simulink library "nodeNetBuoyForce_ul"  (R2020a)
settings: Solver=VariableStepAuto  StartTime=0.0  StopTime=10.0  RelTol=1e-3
settings Model: Creator=mcobb  LastModifiedBy=andre
settings DataIOCC: ReturnWorkspaceOutputs=off
settings DebuggingCC: ArithmeticOperatorsInVariantConditions=warning
settings SFSimCC: CustomCodeUndefinedFunction=UseInterfaceOnly

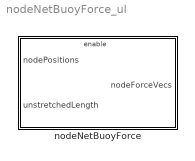
== system nodeNetBuoyForce_ul ==
  nodeNetBuoyForce : Subsystem  mask{fluidDensity=0, tetherDensity=0, diameter=0, gravity=0}
      mask prompts: fluidDensity "Fluid density"; tetherDensity "Tether density"; diameter "Tether diameter"; gravity "Gravitational acceleration"
      settings: MinAlgLoopOccurrences=on

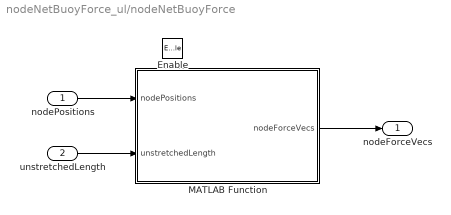
== system nodeNetBuoyForce_ul/nodeNetBuoyForce ==
  nodePositions : Inport
  unstretchedLength : Inport  Port=2
  Enable : EnablePort
  MATLAB Function : MATLAB Function  TreatAsAtomicUnit=on
  nodeForceVecs : Outport  VectorParamsAs1DForOutWhenUnconnected=off
  wires:
  MATLAB Function/1(nodeForceVecs) -> nodeForceVecs/1
  nodePositions/1 -> MATLAB Function/1(nodePositions)
  unstretchedLength/1 -> MATLAB Function/2(unstretchedLength)

== matlab function nodeNetBuoyForce_ul/nodeNetBuoyForce/MATLAB Function ==
  data: nodePositions input; unstretchedLength input; nodeForceVecs output; tetherDensity parameter; fluidDensity parameter; diameter parameter; gravity parameter
function nodeForceVecs  = fcn(...
    nodePositions,unstretchedLength,...
    tetherDensity, fluidDensity, diameter, gravity)

% In this notation, N is the number of nodes

% Length of each link 1xN-1
linkLengths = sqrt(sum(diff(nodePositions,1,2).^2));

% Total length of all links, assuming they're straight lines, scalar
numericalTotalLength = sum(linkLengths);

% Number of links, scalar
numLinks = size(linkLengths,2);

% Total volume based on unspooled length, scalar
analyticalTotalVol  = sum(unstretchedLength)*(pi/4)*diameter^2;

% Total mass, based on unspooled length, scalar
analyticalTotalMass = tetherDensity*analyticalTotalVol;

% Mass of each link, 1xN-1
linkMasses  = analyticalTotalMass*(linkLengths./numericalTotalLength);

% Volume of each link, 1xN-1
linkVolumes = analyticalTotalVol*(linkLengths./numericalTotalLength);

% Net force on the links (buoyancy - gravity) on each link, 3xN-1
linkNetForceVecs = [repmat([0 0]',[1 numLinks]);(-gravity*linkMasses + gravity*fluidDensity*linkVolumes)];

% Net force on the nodes, 3xN
nodeForceVecs = [linkNetForceVecs(:,1) linkNetForceVecs(:,1:end-1)+linkNetForceVecs(:,2:end) linkNetForceVecs(:,end)]/2;


end
